simulink model "ramadan_2021"  (R2020a)
settings: Solver=ode15s  StartTime=0.0  StopTime=20  MaxStep=1e-2  MinStep=1e-20  RelTol=1e-3
StartFcn:
  | tic
StopFcn:
  | toc
  | 
  | 
  | %if GimbalLockFlag
  |  % fprintf(2, 'Almost reached Gimbal Lock of IMU. Simulation stopped.\n')
  | %end
  | 
  | %fprintf('Elapsed time: %4.2f sec (%4.2f%% realtime)\n', a, tout(end)/a*100)
values from neighbouring files (symbols this model uses):
  Balance02 = param(28:31)    [assign_parameters.m]
  Balance13 = param(32:35)    [assign_parameters.m]
  BalanceTrunk = param(22:23)    [assign_parameters.m]
  BalanceTrunkLat = param(24:27)    [assign_parameters.m]
  BasisStim = param(1:11)    [assign_parameters.m]
  CompliantLeg = param(12:14)    [assign_parameters.m]
  CompliantLegLat = param(15)    [assign_parameters.m]
  PreventKneeOverextension = param(16:21)    [assign_parameters.m]
  propulsion = dataset(i,3)    [AssignDataset_BasisPoints.m]    (also in assign_parameters.m = param(43))
  stepDur = dataset(i,2)    [AssignDataset_BasisPoints.m]    (also in assign_parameters.m = param(44))
  Target02 = dataset(i,8:10)    [AssignDataset_BasisPoints.m]    (also in assign_parameters.m = param(36:38))
  Target13 = dataset(i,5:7)    [AssignDataset_BasisPoints.m]    (also in assign_parameters.m = param(39:41))
  Target_lat = param(45)    [assign_parameters.m]
  theta0 = dataset(i,4)    [AssignDataset_BasisPoints.m]    (also in assign_parameters.m = param(42))
  v_init = dataset(i,1)    [AssignDataset_BasisPoints.m]    (also in assign_parameters.m = 1.25)
  WramameiSL_1000 = readmatrix('WSL_1000_Norm_Sigmoid_MSE_cont.csv')    [nms3D_prep.m]
  ZramameiSL_1000 = readmatrix('ZSL_1000_Norm_Sigmoid_MSE_cont.csv')    [nms3D_prep.m]
undefined symbols (not defined in the file or in its folder): ICs, mParams, X, Y, Z
libraries: nesl_utility x110, sm_lib x88, simulink x81, eeGeneralControl x30, robotmaniplib x10, dspinverses x9, robotcorelib x5, dspmathops x3, vrlib x1
(part 1 of 8)
settings Model: SimulationMode=rapid-accelerator  Creator=hgeyer  LastModifiedBy=rachidramadan
settings SolverCC: MinimalZcImpactIntegration=on
settings OptimizationCC: EfficientMapNaN2IntZero=off
settings DebuggingCC: ReadBeforeWriteMsg=DisableAll  WriteAfterWriteMsg=DisableAll  WriteAfterReadMsg=DisableAll  IgnoredZcDiagnostic=none  MultiTaskDSMMsg=none  ArithmeticOperatorsInVariantConditions=warning
settings HardwareCC: TargetBitPerLong=64  TargetBitPerPointer=64  TargetBitPerSizeT=64  TargetBitPerPtrDiffT=64  TargetLongLongMode=on  TargetIntDivRoundTo=Zero  TargetEndianess=LittleEndian  TargetWordSize=64  TargetHWDeviceType=MATLAB Host  ProdEqTarget=off
settings ModelReferenceCC: UpdateModelReferenceTargets=IfOutOfDate
settings SFSimCC: SFSimEcho=off  SimUseLocalCustomCode=off  CustomCodeUndefinedFunction=UseInterfaceOnly
settings CodeAppCC: MaxIdLength=128
settings ConfigComp: CovScope=ReferencedModels
settings SimscapeCC: SimscapeNormalizeSystem=off
settings ExplorerConfigSet: InternalSimMechanicsExplorerSettings="<ExplorerConfiguration><canonicalview>planar_xy</canonicalview><AnimationSetting><BasePlaybackSpeed>1.0</BasePlaybackSpeed><PlaybackSpeedFactor>1.0</PlaybackSpeedFactor></AnimationSetting><TilePanel><TileInfo><Tiles Columns=\"1\" Count=\"1\" Rows=\"1\"><Column Weight=\"1\"/><Row Weight=\"1\"/><Tile Height=\"1\" Width=\"1\" X=\"0\" Y=\"0\"/></Tiles></TileInfo><SceneInfo><SceneViewer><BGColor><R>0.60000002384185791</R><G>0.60000002384185791</G><B>0.60000002384185791</B></BGColor><Camera><DoPerspective>off</DoPerspective><Position><X>0.597774143722594631</X><Y>0.919449529340500282</Y><Z>14.1815791267909113</Z></Position><Center><X>0.597774143722594631</X><Y>0.919449529340500282</Y><Z>3.38181724401920292e-07</Z></Center><Up><X>0</X><Y>1</Y><Z>0</Z></Up><ViewLimDist>1</ViewLimDist><YLim>1.30566284997374105</YLim><XLim>1.60885047805753101</XLim></Camera></SceneViewer></SceneInfo></TilePanel><MechEditorPanel><Cameras/><GfxPanelCameraMap/><VideoCreator><PlaybackSpeedRatio>1.0</PlaybackSpeedRatio><FrameRate>30</FrameRate><VideoFormat>Motion JPEG AVI</VideoFormat><FrameSize>auto</FrameSize></VideoCreator></MechEditorPanel></ExplorerConfiguration>"

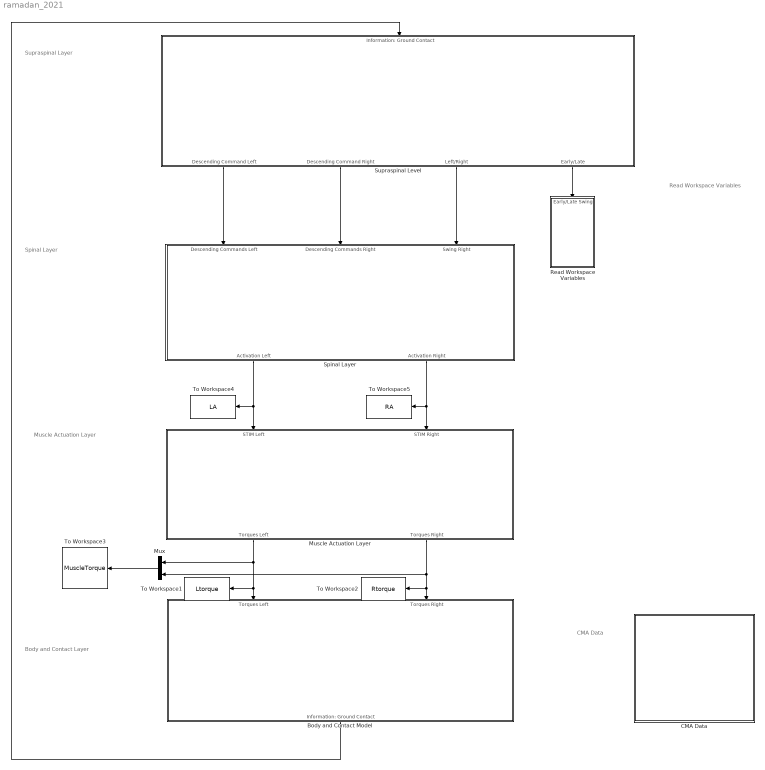
== system ramadan_2021 ==
  note: Spinal Layer
  note: Muscle Actuation Layer
  note: Body and Contact Layer
  note: Supraspinal Layer
  note: CMA Data
  note: Read Workspace Variables
  Body and Contact Model : Subsystem
  CMA Data : Subsystem
  Muscle Actuation Layer : Subsystem
  Mux : Mux  Inputs=2
  Read Workspace Variables : Subsystem
  Spinal Layer : Subsystem
  Supraspinal Level : Subsystem
  To Workspace1 : ToWorkspace  VariableName=Ltorque  SampleTime=-1
      settings: Save2DSignal=2-D array (concatenate along first dimension)
  To Workspace2 : ToWorkspace  VariableName=Rtorque  SampleTime=-1
      settings: Save2DSignal=2-D array (concatenate along first dimension)
  To Workspace3 : ToWorkspace  VariableName=MuscleTorque  SampleTime=-1
      settings: Save2DSignal=2-D array (concatenate along first dimension)
  To Workspace4 : ToWorkspace  VariableName=LA  SampleTime=-1
      settings: Save2DSignal=2-D array (concatenate along first dimension)
  To Workspace5 : ToWorkspace  VariableName=RA  SampleTime=-1
      settings: Save2DSignal=2-D array (concatenate along first dimension)
  wires:
  Spinal Layer/1(Activation Left) -> To Workspace4/1, Muscle Actuation Layer/1(STIM Left)
  Spinal Layer/2(Activation Right) -> To Workspace5/1, Muscle Actuation Layer/2(STIM Right)
  Muscle Actuation Layer/2(Torques Right) -> Mux/2, To Workspace2/1, Body and Contact Model/2(Torques Right)
  Supraspinal Level/1(Descending Command Left) -> Spinal Layer/1(Descending Commands Left)
  Supraspinal Level/2(Descending Command Right) -> Spinal Layer/2(Descending Commands Right)
  Body and Contact Model/1(Information: Ground Contact) -> Supraspinal Level/1(Information: Ground Contact)
  Mux/1 -> To Workspace3/1
  Muscle Actuation Layer/1(Torques Left) -> Mux/1, Body and Contact Model/1(Torques Left), To Workspace1/1
  Supraspinal Level/3(Left/Right) -> Spinal Layer/3(Swing Right)
  Supraspinal Level/4(Early/Late) -> Read Workspace Variables/1(Early/Late Swing)

== system ramadan_2021/Body and Contact Model ==
  note: Rigid Body
  note: Contact Model
  note: Vestibular System
  Torques Left : Inport
  Torques Right : Inport  Port=2
  6-DOF Joint IC : sm_lib/Joints/6-DOF Joint  JointMode=Normal  SenseConstraintForce=off  SenseConstraintForceX=off  SenseConstraintForceY=off  SenseConstraintForceZ=off  SenseConstraintTorque=off  SenseConstraintTorqueX=off  SenseConstraintTorqueY=off  SenseConstraintTorqueZ=off  SenseTotalForce=off  SenseTotalForceX=off  SenseTotalForceY=off  SenseTotalForceZ=off  SenseTotalTorque=off  SenseTotalTorqueX=off  SenseTotalTorqueY=off  SenseTotalTorqueZ=off  CompositeWrenchDir=BaseOnFollower  CompositeWrenchFrame=FollowerFrame  PxEquilibriumPosition=0  PxEquilibriumPositionUnits=m  PxSpringStiffness=0  PxSpringStiffnessUnits=N/m  PxDampingCoefficient=0  PxDampingCoefficientUnits=N/(m/s)  PxTorqueActuationMode=NoTorque  PxMotionActuationMode=ComputedMotion  PxSensePosition=off  PxSenseVelocity=off  PxSenseAcceleration=off  PxSenseTorqueForce=off  PxSenseLowerLimitTorqueForce=off  PxSenseUpperLimitTorqueForce=off  PxLowerLimitSpecify=off  PxLowerLimitBound=-1  PxLowerLimitBoundUnits=m  PxLowerLimitStiffness=1e6  PxLowerLimitStiffnessUnits=N/m  PxLowerLimitDamping=1e3  PxLowerLimitDampingUnits=N/(m/s)  PxLowerLimitTransitionRegionWidth=1e-4  PxLowerLimitTransitionRegionWidthUnits=m  PxUpperLimitSpecify=off  PxUpperLimitBound=1  PxUpperLimitBoundUnits=m  PxUpperLimitStiffness=1e6  PxUpperLimitStiffnessUnits=N/m  PxUpperLimitDamping=1e3  PxUpperLimitDampingUnits=N/(m/s)  PxUpperLimitTransitionRegionWidth=1e-4  PxUpperLimitTransitionRegionWidthUnits=m  PxPositionTargetSpecify=on  PxPositionTargetPriority=High  PxPositionTargetValue=ICs.trunk.x0  PxPositionTargetValueUnits=m  PxVelocityTargetSpecify=on  PxVelocityTargetPriority=High  PxVelocityTargetValue=ICs.trunk.vx0  PxVelocityTargetValueUnits=m/s  PyEquilibriumPosition=0  PyEquilibriumPositionUnits=m  PySpringStiffness=0  PySpringStiffnessUnits=N/m  PyDampingCoefficient=0  PyDampingCoefficientUnits=N/(m/s)  PyTorqueActuationMode=NoTorque  PyMotionActuationMode=ComputedMotion  PySensePosition=off  PySenseVelocity=off  PySenseAcceleration=off  PySenseTorqueForce=off  PySenseLowerLimitTorqueForce=off  PySenseUpperLimitTorqueForce=off  PyLowerLimitSpecify=off  PyLowerLimitBound=-1  PyLowerLimitBoundUnits=m  PyLowerLimitStiffness=1e6  PyLowerLimitStiffnessUnits=N/m  PyLowerLimitDamping=1e3  PyLowerLimitDampingUnits=N/(m/s)  PyLowerLimitTransitionRegionWidth=1e-4  PyLowerLimitTransitionRegionWidthUnits=m  PyUpperLimitSpecify=off  PyUpperLimitBound=1  PyUpperLimitBoundUnits=m  PyUpperLimitStiffness=1e6  PyUpperLimitStiffnessUnits=N/m  PyUpperLimitDamping=1e3  PyUpperLimitDampingUnits=N/(m/s)  PyUpperLimitTransitionRegionWidth=1e-4  PyUpperLimitTransitionRegionWidthUnits=m  PyPositionTargetSpecify=on  PyPositionTargetPriority=High  PyPositionTargetValue=ICs.trunk.y0  PyPositionTargetValueUnits=m  PyVelocityTargetSpecify=off  PyVelocityTargetPriority=High  PyVelocityTargetValue=0  PyVelocityTargetValueUnits=m/s  PzEquilibriumPosition=0  PzEquilibriumPositionUnits=m  PzSpringStiffness=0  PzSpringStiffnessUnits=N/m  PzDampingCoefficient=0  PzDampingCoefficientUnits=N/(m/s)  PzTorqueActuationMode=NoTorque  PzMotionActuationMode=ComputedMotion  PzSensePosition=off  PzSenseVelocity=off  PzSenseAcceleration=off  PzSenseTorqueForce=off  PzSenseLowerLimitTorqueForce=off  PzSenseUpperLimitTorqueForce=off  PzLowerLimitSpecify=off  PzLowerLimitBound=-1  PzLowerLimitBoundUnits=m  PzLowerLimitStiffness=1e6  PzLowerLimitStiffnessUnits=N/m  PzLowerLimitDamping=1e3  PzLowerLimitDampingUnits=N/(m/s)  PzLowerLimitTransitionRegionWidth=1e-4  PzLowerLimitTransitionRegionWidthUnits=m  PzUpperLimitSpecify=off  PzUpperLimitBound=1  PzUpperLimitBoundUnits=m  PzUpperLimitStiffness=1e6  PzUpperLimitStiffnessUnits=N/m  PzUpperLimitDamping=1e3  PzUpperLimitDampingUnits=N/(m/s)  PzUpperLimitTransitionRegionWidth=1e-4  PzUpperLimitTransitionRegionWidthUnits=m  PzPositionTargetSpecify=on  PzPositionTargetPriority=High  PzPositionTargetValue=ICs.trunk.z0  PzPositionTargetValueUnits=m  PzVelocityTargetSpecify=on  PzVelocityTargetPriority=High  PzVelocityTargetValue=ICs.trunk.vz0  PzVelocityTargetValueUnits=m/s  SphDefPosRotationMethod=None  SphDefPosRotationAngleUnits=deg  SphDefPosRotationStandardAxis=+Z  SphDefPosRotationAngle=0.0  SphDefPosRotationArbitraryAxis=[0 0 1]  SphDefPosFollAlignAxisA=+X  SphDefPosBaseAlignAxisA=+Y  SphDefPosFollAlignAxisB=+Y  SphDefPosBaseAlignAxisB=+Z  SphDefPosRotationSequenceAxes=FollowerAxes  SphDefPosRotationSequence=XYX  SphDefPosRotationSequenceAngles=[0 0 0]  SphDefPosRotationSequenceAnglesUnits=deg  SphDefPosRotationMatrix=[1 0 0; 0 1 0; 0 0 1]  SphEqPosRotationMethod=None  SphEqPosRotationAngleUnits=deg  SphEqPosRotationStandardAxis=+Y  SphEqPosRotationAngle=0.0  SphEqPosRotationArbitraryAxis=[0 0 1]  SphEqPosFollAlignAxisA=+X  SphEqPosBaseAlignAxisA=+Y  SphEqPosFollAlignAxisB=+Y  SphEqPosBaseAlignAxisB=+Z  SphEqPosRotationSequenceAxes=FollowerAxes  SphEqPosRotationSequence=XYZ  SphEqPosRotationSequenceAngles=[0 0 -0.3]  SphEqPosRotationSequenceAnglesUnits=rad  SphEqPosRotationMatrix=[1 0 0; 0 1 0; 0 0 1]  SphSpringStiffness=0  SphSpringStiffnessUnits=N*m/deg  SphDampingCoefficient=0  SphDampingCoefficientUnits=N*m/(deg/s)  SphActuateTorqueX=off  SphActuateTorqueY=off  SphActuateTorqueZ=off  SphActuateTorque=on  SphTorqueActuationMode=NoTorque  SphMotionActuationMode=ComputedMotion  SphActuationFrame=BaseFrame  SphSensePosition=off  SphSenseVelocityX=off  SphSenseVelocityY=off  SphSenseVelocityZ=off  SphSenseVelocity=off  SphSenseAccelerationX=off  SphSenseAccelerationY=off  SphSenseAccelerationZ=off  SphSenseAcceleration=off  SphSenseTorqueX=off  SphSenseTorqueY=off  SphSenseTorqueZ=off  SphSenseTorqueForce=off  SphSenseLowerLimitTorqueMag=off  SphSenseUpperLimitTorqueMag=off  SphSensingFrame=BaseFrame  SphLowerLimitSpecify=off  SphLowerLimitBound=15  SphLowerLimitBoundUnits=deg  SphLowerLimitStiffness=1e4  SphLowerLimitStiffnessUnits=N*m/deg  SphLowerLimitDamping=10  SphLowerLimitDampingUnits=N*m/(deg/s)  SphLowerLimitTransitionRegionWidth=0.1  SphLowerLimitTransitionRegionWidthUnits=deg  SphUpperLimitSpecify=off  SphUpperLimitBound=45  SphUpperLimitBoundUnits=deg  SphUpperLimitStiffness=1e4  SphUpperLimitStiffnessUnits=N*m/deg  SphUpperLimitDamping=10  SphUpperLimitDampingUnits=N*m/(deg/s)  SphUpperLimitTransitionRegionWidth=0.1  SphUpperLimitTransitionRegionWidthUnits=deg  SphPositionTargetRotationMethod=RotationSequence  SphPositionTargetRotationAngleUnits=deg  SphPositionTargetRotationStandardAxis=+Z  SphPositionTargetRotationAngle=0.0  SphPositionTargetRotationArbitraryAxis=[0 0 1]  SphPositionTargetFollAlignAxisA=+X  SphPositionTargetBaseAlignAxisA=+Y  SphPositionTargetFollAlignAxisB=+Y  SphPositionTargetBaseAlignAxisB=+Z  SphPositionTargetRotationSequenceAxes=BaseAxes  SphPositionTargetRotationSequence=XZY  SphPositionTargetRotationSequenceAngles=[ICs.trunk.qR0 ICs.trunk.qP0 ICs.trunk.qY0 ]  SphPositionTargetRotationSequenceAnglesUnits=rad  SphPositionTargetRotationMatrix=[1 0 0; 0 1 0; 0 0 1]  SphPositionTargetSpecify=on  SphPositionTargetPriority=High  SphVelocityTargetValue=[ICs.trunk.qR0 ICs.trunk.qP0 ICs.trunk.qY0 ]  SphVelocityTargetValueUnits=deg/s  SphVelocityTargetSpecify=on  SphVelocityTargetPriority=High  SphVelocityTargetInFollowerFrame=on
  Clock : Clock
  Compare To Constant : simulink/Logic and Bit Operations/Compare To Constant  relop=<=  const=0.05  OutDataTypeStr=boolean
  Constant : Constant  Value=0
  External Force and Torque : sm_lib/Forces and Torques/External Force and Torque  ForceResolutionFrame=AttachedFrame  EnableForceX=on  EnableForceY=off  EnableForceZ=off  EnableForce=off  TorqueResolutionFrame=AttachedFrame  EnableTorqueX=off  EnableTorqueY=off  EnableTorqueZ=off  EnableTorque=off
  L Leg : Subsystem
  Minus : Sum  Inputs=-+
  PID Controller : simulink/Continuous/PID Controller  Controller=P  Form=Parallel  TimeDomain=Continuous-time  UseExternalTs=off  SampleTime=-1  IntegratorMethod=Forward Euler  FilterMethod=Forward Euler  ControllerParametersSource=internal  P=7000  I=1  D=0  UseFilter=on  N=100  TunerSelectOption=Transfer Function Based (PID Tuner App)  ZeroCross=off  InitialConditionSource=internal  InitialConditionForIntegrator=0  InitialConditionForFilter=0  DifferentiatorICPrevScaledInput=0  ExternalReset=none  TrackingMode=off  Kt=1  LimitOutput=off  UpperSaturationLimit=inf  LowerSaturationLimit=-inf  LinearizeAsGain=on  AntiWindupMode=none  Kb=1  POutMin=[]  POutMax=[]  IOutMin=[]  IOutMax=[]  DOutMin=[]  DOutMax=[]  NOutMin=[]  NOutMax=[]  SumOutMin=[]  SumOutMax=[]  SaturationOutMin=[]  SaturationOutMax=[]  PParamMin=[]  PParamMax=[]  IParamMin=[]  IParamMax=[]  DParamMin=[]  DParamMax=[]  NParamMin=[]  NParamMax=[]  KbParamMin=[]  KbParamMax=[]  KtParamMin=[]  KtParamMax=[]  KbOutMin=[]  KbOutMax=[]  KtOutMin=[]  KtOutMax=[]  IntegratorOutMin=[]  IntegratorOutMax=[]  FilterOutMin=[]  FilterOutMax=[]  SumI1OutMin=[]  SumI1OutMax=[]  SumI2OutMin=[]  SumI2OutMax=[]  SumI3OutMin=[]  SumI3OutMax=[]  SumI4OutMin=[]  SumI4OutMax=[]  SumDOutMin=[]  SumDOutMax=[]  DifferentiatorOutMin=[]  DifferentiatorOutMax=[]  FilterDiffOutCoefMin=[]  FilterDiffOutCoefMax=[]  ReciprocalOutMin=[]  ReciprocalOutMax=[]  SumDenOutMin=[]  SumDenOutMax=[]  SumNumOutMin=[]  SumNumOutMax=[]  DivideOutMin=[]  DivideOutMax=[]  UdiffTsProdOutMin=[]  UdiffTsProdOutMax=[]  NTsProdOutMin=[]  NTsProdOutMax=[]  UintegralTsProdOutMin=[]  UintegralTsProdOutMax=[]  UngainTsProdOutMin=[]  UngainTsProdOutMax=[]  IntegratorContinuousStateAttributes=''  IntegratorStateMustResolveToSignalObject=off  IntegratorRTWStateStorageClass=Auto  FilterContinuousStateAttributes=''  FilterStateMustResolveToSignalObject=off  FilterRTWStateStorageClass=Auto  ParallelPVariant=InternalParameters  IdealPVariant=Disabled  IVariant=Disabled  DVariant=Disabled  IntegratorVariant=Disabled  SatVariant=Disabled  AWVariant=Disabled  PCopyVariant=Disabled  TRVariant=Disabled  FdbkBlocksVariant=Forward  IdealPFdbkVariant=Disabled  SatFdbkVariant=Disabled  DerivativeFilterVariant=Disabled  NVariant=Disabled  NCopyVariant=Disabled_SignalSpec  FilterICVariant=Disabled  IntegratorICVariant=Disabled  ExternalResetVariant=Disabled  TRSumVariant=Passthrough  SumFdbkVariant=Disabled  SumVariant=Passthrough_P  TsampFilterVariant=InternalTs  TsampNgainVariant=Passthrough  TsampIntegralVariant=Disabled_SignalSpec
  R Leg : Subsystem
  Selector : Selector  InputPortWidth=3  IndexOptions=Index vector (dialog)  Indices=[1]  OutputSizes=1
  Sensor Left Ankle : Subsystem
  Sensor Left Ankle1 : Subsystem
  Simulink-PS Converter : nesl_utility/Simulink-PS Converter  PhysicalDomain=network_engine_domain  SubClassName=ps_input  LeftPortType=input  RightPortType=output  PseudoPeriodic=off  Frequencies=[]  NoiseDistribution=none  NoiseParameters=[]  Unit=1  AffineConversion=off  FilteringAndDerivatives=provide  SimscapeFilterOrder=1  InputFilterTimeConstant=0.001  UdotUserProvided=0
  Subsystem : Subsystem
  Switch : Switch  Criteria=u2 > Threshold
  Terminator : Terminator
  Terminator1 : Terminator
  To Workspace1 : ToWorkspace  VariableName=Rlegq  SampleTime=-1
      settings: Save2DSignal=2-D array (concatenate along first dimension)
  To Workspace3 : ToWorkspace  VariableName=Llegq  SampleTime=-1
      settings: Save2DSignal=2-D array (concatenate along first dimension)
  Trunk (floating base) : Subsystem
  Vestibular System : Subsystem
  World Frame : Subsystem
  Information: Ground Contact : Outport
  tag scope: LHL=global, LHR=global, Llegddq=global, Llegdq=global, Llegq=global, Rlegddq=global, Rlegdq=global, Rlegq=global
  wires:
  R Leg/4("Joint Velocities Right [rad/s] ") -> [Rlegdq]
  R Leg/5(Joint Accelerations Right [rad/s^2]) -> [Rlegddq]
  R Leg/3(Joint Angles Right [rad]) -> To Workspace1/1, [Rlegq]
  L Leg/3(Joint Angles Left [rad]) -> To Workspace3/1, [Llegq]
  L Leg/5(Joint Accelerations Left [rad/s^2]) -> [Llegddq]
  L Leg/4("Joint Velocities Left [rad/s] ") -> [Llegdq]
  R Leg/2(Position Right Ankle [m]) -> Vestibular System/1(Ankle Position Right [m])
  L Leg/2(" Position Left Ankle [m]") -> Vestibular System/2(Ankle Position Left [m])
  Subsystem/1(Information: Ground Contact) -> Information: Ground Contact/1
  L Leg/1(Rotation Matrix Left Knee (world)) -> Terminator/1
  R Leg/1(Rotation Matrix Right Knee (World)) -> Terminator1/1
  Torques Right/1 -> R Leg/1(Torques [Nm])
  Torques Left/1 -> L Leg/1(Torques [Nm])
  Sensor Left Ankle/1(Position [m]) -> [LHL]
  Sensor Left Ankle1/1(Position [m]) -> [LHR]
  [CoM_Velocity] -> Selector/1
  Selector/1 -> Minus/1
  [v_init] -> Minus/2
  Minus/1 -> PID Controller/1
  PID Controller/1 -> Switch/1
  Constant/1 -> Switch/3
  Clock/1 -> Compare To Constant/1
  Compare To Constant/1 -> Switch/2
  Switch/1 -> Simulink-PS Converter/1
  connections:
  Trunk (floating base)/RConn1 -- Vestibular System/LConn3 -- L Leg/LConn1
  World Frame/RConn1 -- Subsystem/LConn1 -- 6-DOF Joint IC/LConn1
  L Leg/RConn1 -- Subsystem/RConn1
  L Leg/RConn2 -- Sensor Left Ankle/LConn1 -- Subsystem/RConn2
  L Leg/RConn3 -- Subsystem/RConn3
  L Leg/RConn4 -- Subsystem/RConn4
  R Leg/RConn3 -- Subsystem/RConn7
  R Leg/RConn4 -- Subsystem/RConn8
  Vestibular System/LConn2 -- R Leg/LConn1 -- Trunk (floating base)/RConn2
  6-DOF Joint IC/RConn1 -- Vestibular System/LConn1 -- Trunk (floating base)/LConn1 -- External Force and Torque/RConn1
  Subsystem/RConn6 -- Sensor Left Ankle1/LConn1 -- R Leg/RConn1
  R Leg/RConn2 -- Subsystem/RConn5
  External Force and Torque/LConn1 -- Simulink-PS Converter/RConn1

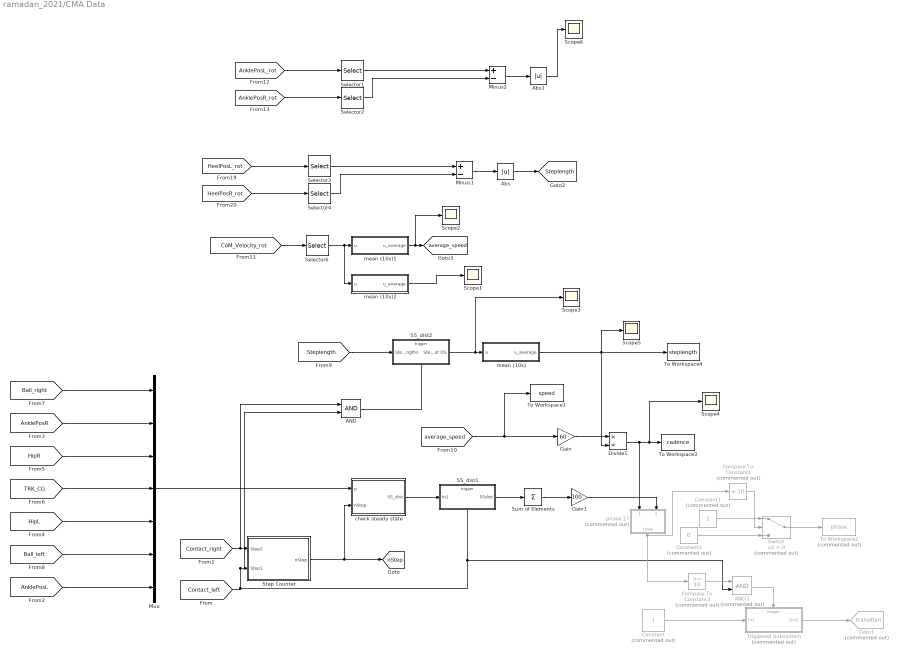
== system ramadan_2021/CMA Data ==
  AND : Logic  AllPortsSameDT=off  OutDataTypeStr=boolean
  AND3 : Logic  Commented=on  AllPortsSameDT=off  OutDataTypeStr=boolean
  Abs : Abs  ZeroCross=off
  Abs1 : Abs  ZeroCross=off
  Compare To Constant1 : simulink/Logic and Bit Operations/Compare To Constant  Commented=on  relop=>  const=10  OutDataTypeStr=boolean
  Compare To Constant3 : simulink/Logic and Bit Operations/Compare To Constant  Commented=on  relop=>=  const=10  OutDataTypeStr=boolean
  Constant : Constant  Commented=on  VectorParams1D=off  SampleTime=-1
  Constant1 : Constant  Commented=on
  Constant2 : Constant  Commented=on  Value=0
  Divide1 : Product  Inputs=*/
  Gain : Gain  Gain=60
  Gain1 : Gain  Gain=100
  Goto1 : Goto  Commented=on  GotoTag=transition  TagVisibility=global
  Minus1 : Sum  Inputs=+-
  Minus2 : Sum  Inputs=+-
  Mux : Mux  Inputs=7
  SS_dist1 : Subsystem  TreatAsAtomicUnit=on
  SS_dist2 : Subsystem  TreatAsAtomicUnit=on
  Scope{1..6} (6 alike) : Scope
  Selector{1..4,6} (5 alike) : Selector  InputPortWidth=3  IndexOptions=Index vector (dialog)  Indices=[1]  OutputSizes=1
  Step Counter : Subsystem
  Sum of Elements : Sum  Inputs=+
  Switch : Switch  Commented=on  Criteria=u2 > Threshold
  To Workspace1 : ToWorkspace  VariableName=speed  SampleTime=-1
      settings: Save2DSignal=2-D array (concatenate along first dimension)
  To Workspace2 : ToWorkspace  Commented=on  VariableName=phase  SampleTime=-1
      settings: Save2DSignal=2-D array (concatenate along first dimension)
  To Workspace3 : ToWorkspace  VariableName=cadence  SampleTime=-1
      settings: Save2DSignal=2-D array (concatenate along first dimension)
  To Workspace4 : ToWorkspace  VariableName=steplength  SampleTime=-1
      settings: Save2DSignal=2-D array (concatenate along first dimension)
  Triggered Subsystem : Subsystem  Commented=on  TreatAsAtomicUnit=on
  check steady state : Subsystem
  mean (10s) : Subsystem
  mean (10s)1 : Subsystem
  mean (10s)2 : Subsystem
  phase 1? : Subsystem  Commented=on
  tag scope: Steplength=global, average_speed=global, nStep=global
  wires:
  Step Counter/1(nStep) -> check steady state/2(nStep), [nStep]
  [Contact_left] -> AND/2, Step Counter/2(Step1), SS_dist1/Trigger, AND3/2
  [Contact_right] -> AND/1, Step Counter/1(Step2)
  [Ball_right] -> Mux/1
  [AnklePosR] -> Mux/2
  [HipR] -> Mux/3
  [TRK_CG] -> Mux/4
  [HipL] -> Mux/5
  [Ball_left] -> Mux/6
  [AnklePosL] -> Mux/7
  Mux/1 -> check steady state/1(p)
  check steady state/1(SS_dist) -> SS_dist1/1(In1)
  [Steplength] -> SS_dist2/1(Steplengths)
  SS_dist2/1(Steplength at DS) -> Scope3/1, mean (10s)/1(u)
  AND/1 -> SS_dist2/Trigger
  mean (10s)/1(u_average) -> Divide1/2, To Workspace4/1, Scope5/1
  [average_speed] -> To Workspace1/1, Gain/1
  Divide1/1 -> Scope4/1, To Workspace3/1, phase 1?/1(cadence)
  Gain/1 -> Divide1/1
  SS_dist1/1(SSdist) -> Sum of Elements/1
  Sum of Elements/1 -> Gain1/1
  Compare To Constant3/1 -> AND3/1
  AND3/1 -> Triggered Subsystem/Trigger
  Triggered Subsystem/1(Out1) -> Goto1/1
  Constant/1 -> Triggered Subsystem/1(In1)
  Gain1/1 -> phase 1?/2(stability)
  phase 1?/1(time) -> Compare To Constant1/1, Compare To Constant3/1
  Constant1/1 -> Switch/1
  Constant2/1 -> Switch/3
  Switch/1 -> To Workspace2/1
  Compare To Constant1/1 -> Switch/2
  Selector3/1 -> Minus1/1
  [HeelPosL_rot] -> Selector3/1
  Selector4/1 -> Minus1/2
  [HeelPosR_rot] -> Selector4/1
  Minus1/1 -> Abs/1
  Abs/1 -> [Steplength]
  [CoM_Velocity_rot] -> Selector6/1
  mean (10s)1/1(u_average) -> Scope2/1, [average_speed]
  Selector6/1 -> mean (10s)2/1(u), mean (10s)1/1(u)
  Selector2/1 -> Minus2/2
  Abs1/1 -> Scope6/1
  [AnklePosL_rot] -> Selector1/1
  [AnklePosR_rot] -> Selector2/1
  Selector1/1 -> Minus2/1
  Minus2/1 -> Abs1/1
  mean (10s)2/1(u_average) -> Scope1/1

== system ramadan_2021/Muscle Actuation Layer ==
  note: Muscle Actuation Layer
  STIM Left : Inport
  STIM Right : Inport  Port=2
  Muscles Left : Subsystem
  Muscles Right : Subsystem
  Mux : Mux
  Mux1 : Mux
  Torques Left : Outport
  Torques Right : Outport  Port=2
  tag scope: BalanceTorqueLeft=global, stance_torque_left_norm=global, stance_torque_right_norm=global
  wires:
  STIM Left/1 -> Muscles Left/1(STIM Left)
  STIM Right/1 -> Muscles Right/1(STIM Right)
  Muscles Left/1(tauHipPitchL) -> Mux/1
  Muscles Left/2(tauHipRollL) -> Mux/2
  Muscles Right/1(tauHipPitchR) -> Mux1/1
  Muscles Right/2(tauHipRollR) -> Mux1/2
  Muscles Left/4(tauHipAnkleL) -> Mux/4
  Muscles Right/3(tauKneeR) -> Mux1/3
  Muscles Left/3(tauKneeL) -> Mux/3
  Muscles Right/4(tauHipAnkleR) -> Mux1/4
  Mux/1 -> Torques Left/1
  Mux1/1 -> Torques Right/1
  Muscles Right/5(Leg Torque) -> [stance_torque_right_norm]
  Muscles Left/5("Leg Torque ") -> [stance_torque_left_norm]

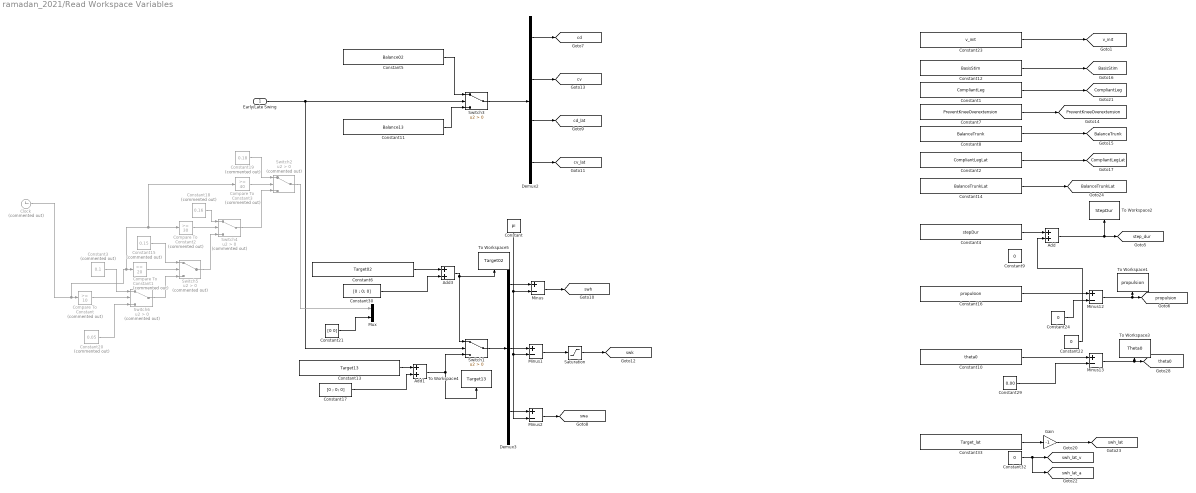
== system ramadan_2021/Read Workspace Variables ==
  Early/Late Swing : Inport
  Add : Sum
  Add1 : Sum
  Add3 : Sum
  Clock : Clock  Commented=on
  Compare To Constant : simulink/Logic and Bit Operations/Compare To Constant  Commented=on  relop=>=  const=10  OutDataTypeStr=boolean
  Compare To Constant1 : simulink/Logic and Bit Operations/Compare To Constant  Commented=on  relop=>=  const=20  OutDataTypeStr=boolean
  Compare To Constant2 : simulink/Logic and Bit Operations/Compare To Constant  Commented=on  relop=>=  const=30  OutDataTypeStr=boolean
  Compare To Constant3 : simulink/Logic and Bit Operations/Compare To Constant  Commented=on  relop=>=  const=40  OutDataTypeStr=boolean
  Constant : Constant  Value=pi
  Constant1 : Constant  Value=CompliantLeg
  Constant10 : Constant  Value=theta0
  Constant11 : Constant  Value=Balance13
  Constant12 : Constant  Value=BasisStim
  Constant13 : Constant  Value=Target13
  Constant14 : Constant  Value=BalanceTrunkLat
  Constant15 : Constant  Commented=on  Value=0.15
  Constant16 : Constant  Value=propulsion
  Constant17 : Constant  Value=[0 ; 0; 0]
  Constant18 : Constant  Commented=on  Value=0.16
  Constant19 : Constant  Commented=on  Value=0.18
  Constant2 : Constant  Value=CompliantLegLat
  Constant20 : Constant  Commented=on  Value=0.05
  Constant21 : Constant  Value=[0 0]
  Constant{9,22,24,32} (4 alike) : Constant  Value=0
  Constant23 : Constant  Value=v_init
  Constant29 : Constant  Value=0.00
  Constant3 : Constant  Commented=on  Value=0.1
  Constant30 : Constant  Value=[0 ; 0; 0]
  Constant33 : Constant  Value=Target_lat
  Constant4 : Constant  Value=stepDur
  Constant5 : Constant  Value=Balance02
  Constant6 : Constant  Value=Target02
  Constant7 : Constant  Value=PreventKneeOverextension
  Constant8 : Constant  Value=BalanceTrunk
  Demux2 : Demux
  Demux3 : Demux  Outputs=3
  Gain : Gain  Gain=-1
  Minus{,1..2,12..13} (5 alike) : Sum  Inputs=+-
  Mux : Mux  Inputs=2
  Saturation : Saturate  UpperLimit=pi  LowerLimit=0  ZeroCross=off
  Switch1 : Switch  Criteria=u2 > Threshold
  Switch{2,4..6} (4 alike) : Switch  Commented=on  Criteria=u2 > Threshold
  Switch3 : Switch  Criteria=u2 > Threshold  ZeroCross=off
  To Workspace1 : ToWorkspace  VariableName=propulsion  SampleTime=-1
      settings: Save2DSignal=2-D array (concatenate along first dimension)
  To Workspace2 : ToWorkspace  VariableName=StepDur  SampleTime=-1
      settings: Save2DSignal=2-D array (concatenate along first dimension)
  To Workspace3 : ToWorkspace  VariableName=Theta0  SampleTime=-1
      settings: Save2DSignal=2-D array (concatenate along first dimension)
  To Workspace4 : ToWorkspace  VariableName=Target13  SampleTime=-1
      settings: Save2DSignal=2-D array (concatenate along first dimension)
  To Workspace5 : ToWorkspace  VariableName=Target02  SampleTime=-1
      settings: Save2DSignal=2-D array (concatenate along first dimension)
  tag scope: BalanceTrunk=global, BalanceTrunkLat=global, BasisStim=global, CompliantLeg=global, CompliantLegLat=global, PreventKneeOverextension=global, cd=global, cd_lat=global, cv=global, cv_lat=global, propulsion=global, step_dur=global, swa=global, swh=global, swh_lat=global, swh_lat_a=global, swh_lat_v=global, swk=global, theta0=global, v_init=global
  wires:
  Constant1/1 -> [CompliantLeg]
  Constant8/1 -> [BalanceTrunk]
  Constant12/1 -> [BasisStim]
  Constant7/1 -> [PreventKneeOverextension]
  Switch1/1 -> Demux3/1
  Demux2/3 -> [cd_lat]
  Demux2/2 -> [cv]
  Switch3/1 -> Demux2/1
  Demux2/4 -> [cv_lat]
  Demux2/1 -> [cd]
  Constant2/1 -> [CompliantLegLat]
  Minus/1 -> [swh]
  Demux3/1 -> Minus/1
  Minus1/1 -> Saturation/1
  Demux3/2 -> Minus1/1
  Minus2/1 -> [swa]
  Demux3/3 -> Minus2/1
  Constant/1 -> Minus/2, Minus1/2, Minus2/2
  Constant14/1 -> [BalanceTrunkLat]
  Early/Late Swing/1 -> Switch1/2, Switch3/2
  Constant33/1 -> Gain/1
  Saturation/1 -> [swk]
  Minus12/1 -> To Workspace1/1, [propulsion]
  Constant16/1 -> Minus12/1
  Constant4/1 -> Add/1
  Add/1 -> [step_dur], To Workspace2/1
  Constant13/1 -> Add1/1
  Add1/1 -> To Workspace4/1, Switch1/3
  Constant17/1 -> Add1/2
  Constant11/1 -> Switch3/3
  Constant10/1 -> Minus13/1
  Minus13/1 -> To Workspace3/1, [theta0]
  Constant6/1 -> Add3/1
  Add3/1 -> To Workspace5/1, Switch1/1
  Constant5/1 -> Switch3/1
  Constant32/1 -> [swh_lat_a], [swh_lat_v]
  Gain/1 -> [swh_lat]
  Compare To Constant3/1 -> Switch2/2
  Constant19/1 -> Switch2/1
  Switch4/1 -> Switch2/3
  Compare To Constant2/1 -> Switch4/2
  Constant18/1 -> Switch4/1
  Switch5/1 -> Switch4/3
  Compare To Constant1/1 -> Switch5/2
  Constant15/1 -> Switch5/1
  Switch6/1 -> Switch5/3
  Constant3/1 -> Switch6/1
  Compare To Constant/1 -> Switch6/2
  Constant20/1 -> Switch6/3
  Clock/1 -> Compare To Constant3/1, Compare To Constant2/1, Compare To Constant1/1, Compare To Constant/1
  Switch2/1 -> Mux/1
  Constant21/1 -> Mux/2
  Constant22/1 -> Add/2
  Constant29/1 -> Minus13/2
  Constant24/1 -> Minus12/2
  Constant30/1 -> Add3/2
  Constant23/1 -> [v_init]

== system ramadan_2021/Spinal Layer ==
  Descending Commands Left : Inport
  Descending Commands Right : Inport  Port=2
  Swing Right : Inport  Port=3
  Add1 : Sum
  Add2 : Sum
  Saturation1 : Saturate  UpperLimit=1  LowerLimit=0.001  ZeroCross=off
  Saturation2 : Saturate  UpperLimit=1  LowerLimit=0.001  ZeroCross=off
  Scope{,1..3} (4 alike) : Scope
  Stance Leg Control Left : Subsystem
  Stance Leg Control Right : Subsystem
  Stretch Reflex for Swing Leg Control : Subsystem
  Switch : Switch  Criteria=u2 > Threshold
  Switch1 : Switch  Criteria=u2 > Threshold
  Activation Left : Outport
  Activation Right : Outport  Port=2
  wires:
  Descending Commands Right/1 -> Stretch Reflex for Swing Leg Control/2(Descending Commands Right)
  Descending Commands Left/1 -> Stretch Reflex for Swing Leg Control/1(Descending Commands Left)
  Swing Right/1 -> Switch/2, Stance Leg Control Right/1(Left/Right), Stance Leg Control Left/1(Left/Right), Switch1/2
  Stance Leg Control Left/1(Activation Left) -> Scope1/1, Add1/2
  Stance Leg Control Right/1(Activation Right) -> Scope3/1, Add2/2
  Switch1/1 -> Saturation1/1
  Switch/1 -> Saturation2/1
  Add1/1 -> Switch1/1
  Add2/1 -> Switch/3
  Saturation1/1 -> Activation Left/1
  Saturation2/1 -> Activation Right/1
  Stretch Reflex for Swing Leg Control/2(Activation Right) -> Add2/1, Switch/1, Scope2/1
  Stretch Reflex for Swing Leg Control/1(Activation Left) -> Scope/1, Add1/1, Switch1/3

== system ramadan_2021/Supraspinal Level ==
  note: Finite State Machine
  note: Computing Descending Commands for Swing Leg Control
  Information: Ground Contact : Inport
  Early/ Late : Logic  Operator=OR  AllPortsSameDT=off  OutDataTypeStr=boolean
  Finite State Machine : Subsystem
  Left/ Right : Logic  Operator=OR  AllPortsSameDT=off  OutDataTypeStr=boolean
  Subsystem : Subsystem
  Terminator : Terminator
  To Workspace1 : ToWorkspace  VariableName=LateRight  SampleTime=-1
      settings: Save2DSignal=2-D array (concatenate along first dimension)
  To Workspace2 : ToWorkspace  VariableName=EarlyRight  SampleTime=-1
      settings: Save2DSignal=2-D array (concatenate along first dimension)
  To Workspace3 : ToWorkspace  VariableName=EarlyLeft  SampleTime=-1
      settings: Save2DSignal=2-D array (concatenate along first dimension)
  To Workspace4 : ToWorkspace  VariableName=Contact  SampleTime=-1
      settings: Save2DSignal=2-D array (concatenate along first dimension)
  Descending Command Left : Outport
  Descending Command Right : Outport  Port=2
  Left/Right : Outport  Port=3
  Early/Late : Outport  Port=4
  wires:
  Finite State Machine/3(Early Left Swing) -> To Workspace3/1, Early/ Late/2
  Finite State Machine/1(Early Right Swing) -> To Workspace2/1, Left/ Right/1, Early/ Late/1
  Finite State Machine/4(Late Left Swing) -> Terminator/1
  Finite State Machine/2(Late Right Swing) -> To Workspace1/1, Left/ Right/2
  Early/ Late/1 -> Subsystem/1(Early/Late Swing), Early/Late/1
  Information: Ground Contact/1 -> To Workspace4/1, Finite State Machine/1(Information: Ground Contact)
  Subsystem/1(Descending Command Left) -> Descending Command Left/1
  Subsystem/2(Descending Command Right) -> Descending Command Right/1
  Left/ Right/1 -> Subsystem/2(Swing Right), Left/Right/1
